simulink model "Direct_Force_Pose_NMPC"  (R2021a)
settings: Solver=ode4  StartTime=0.0  StopTime=10  FixedStep=0.001  MaxStep=0.2  RelTol=1e-3
settings Model: Creator=Hameed  LastModifiedBy=Hameed

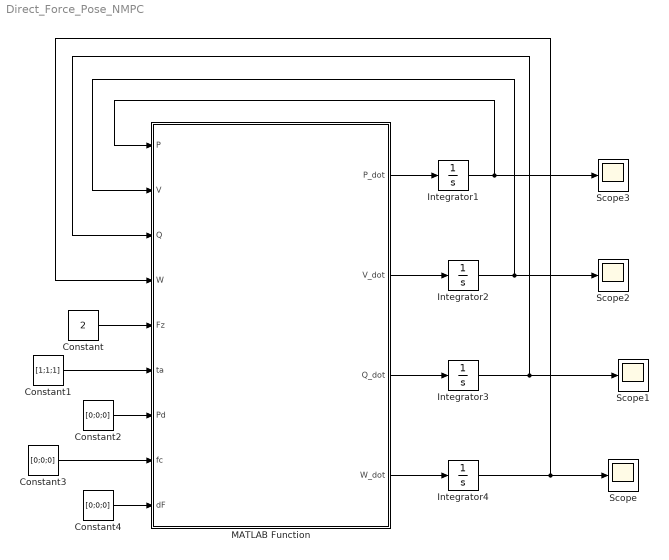
== system Direct_Force_Pose_NMPC ==
  Constant : Constant  Value=2
  Constant1 : Constant  Value=[1;1;1]  VectorParams1D=off
  Constant2 : Constant  Value=[0;0;0]  VectorParams1D=off
  Constant3 : Constant  Value=[0;0;0]  VectorParams1D=off
  Constant4 : Constant  Value=[0;0;0]  VectorParams1D=off
  Integrator1 : Integrator  InitialCondition=[0;0;0]
  Integrator2 : Integrator  InitialCondition=[0;0;0]
  Integrator3 : Integrator  InitialCondition=[0;0;0;0]
  Integrator4 : Integrator  InitialCondition=[0;0;0]
  MATLAB Function : MATLAB Function  TreatAsAtomicUnit=on
  Scope{,1..3} (4 alike) : Scope
  wires:
  MATLAB Function/1(P_dot) -> Integrator1/1
  Integrator4/1 -> Scope/1, MATLAB Function/4(W)
  Integrator2/1 -> Scope2/1, MATLAB Function/2(V)
  MATLAB Function/4(W_dot) -> Integrator4/1
  Integrator3/1 -> MATLAB Function/3(Q), Scope1/1
  Integrator1/1 -> Scope3/1, MATLAB Function/1(P)
  MATLAB Function/3(Q_dot) -> Integrator3/1
  MATLAB Function/2(V_dot) -> Integrator2/1
  Constant/1 -> MATLAB Function/5(Fz)
  Constant2/1 -> MATLAB Function/7(Pd)
  Constant1/1 -> MATLAB Function/6(ta)
  Constant3/1 -> MATLAB Function/8(fc)
  Constant4/1 -> MATLAB Function/9(dF)

== matlab function Direct_Force_Pose_NMPC/MATLAB Function ==
  data: P input; P_dot output; V input; Q input; W input; V_dot output; Q_dot output; W_dot output; Fz input; ta input; Pd input; fc input; dF input
function [P_dot,V_dot,Q_dot,W_dot]= fcn(P,V,Q,W,Fz,ta,Pd,fc,dF)
clc
m=5;
Rz=[cos(Q(4)) sin(Q(4)) 0;-sin(Q(4)) cos(Q(4)) 0;0 0 1];
Rx=[1 0 0;0 cos(Q(2)) sin(Q(2));0 -sin(Q(2)) cos(Q(2))];
Ry=[cos(Q(3)) 0 sin(Q(3));0 1 0;-sin(Q(3)) 0 cos(Q(3))];
Rs=Rz*Rx*Ry;
%lambda=L;
L=1;
%L=0;
Rd=[1 0 0;0 1 0;0 0 1-L];
SL=Rs*Rd*transpose(Rs);
%V=[Vx;Vy;Vz];
Rb=Rz;
fa=[0;0;Fz];

g=9.8;
ab=(m^-1)*((Rb*fa)+(L*fc)+dF)+[0;0;g];

P_dot=SL*V;
%rT=[rx;ry;rz];
rT=P-Pd;
%W=[Wx;Wy;Wz];


Q_dot=(1/2)*Q.*[0;W];

Ixx=1;
Iyy=1;
Izz=1;
J=[Ixx 0 0;0 Iyy 0;0 0 Izz];
%ta=[tx;ty;tz];
h=J*W;
rcom=[0;0;0];
h1=transpose(Rb)*[0;0;m*g];
dT=[0;0;0];
h2=L*transpose(Rb)*fc;
W_dot=(inv(J))*(ta-cross(W,h)+cross(rcom,h1)+cross(rT,h2)+dT);
V_dot=SL*((ab)+Rb*(cross(W_dot,rT)+(cross(W,cross(W,rT)))));
